simulink model "sm_stewart_platform"  (R2019b)
settings: Solver=ode45  StartTime=0.0  StopTime=450  MaxStep=0.2  RelTol=1e-3  EnableMultiTasking=on
model workspace (MAT data in the model file):
  g_density = 5
values from neighbouring files (symbols this model uses):
  B = base_points.Data(:,:,1)    [run_this_for_sim.m]
  base_radius = 0.75*100    (= 75)    [run_this_for_sim.m]
  desired_max_angle = 10    [run_this_for_sim.m]
  desired_max_x = 0.05    [run_this_for_sim.m]
  desired_max_y = desired_max_x    (= 0.05)    [run_this_for_sim.m]
  desired_max_z = 0.05    [run_this_for_sim.m]
  initial_integral_force = 200    [run_this_for_sim.m]
  leg_max = leg_min+0.3    (= 1.322)    [run_this_for_sim.m]
  leg_min = 1.022    [run_this_for_sim.m]
  leg_thickness = 75/1000    (= 0.075)    [run_this_for_sim.m]
  lower_leg_length = upper_leg_length    (= 0.511)    [run_this_for_sim.m]
  max_velocity = 0.15    [run_this_for_sim.m]
  P = platform_points.Data(:,:,1)    [run_this_for_sim.m]
  platform_radius = 0.75*base_radius    (= 56.25)    [run_this_for_sim.m]
  platform_thickness = 0.1/8    (= 0.0125)    [run_this_for_sim.m]
  trajectory_smoothing = 1/1.5    (= 0.666666666667)    [run_this_for_sim.m]
  upper_leg_length = dead_length/2    (= 0.511)    [run_this_for_sim.m]
  work_height = 1.2*100    (= 120)    [run_this_for_sim.m]
undefined symbols (not defined in the file or in its folder): nom_length, X, Z
libraries: sp_lib x18, nesl_utility x11, sm_lib x9, simulink x2
(part 9 of 10)

== system sm_stewart_platform/Stewart Platform System/Manipulator/Platform ==
  Bus Creator : BusCreator  Inputs=6
  Coupling Transform : sm_lib/Frames and Transforms/Rigid Transform  TranslationMethod=StandardAxis  TranslationStandardOffset=(1 - 2 * kind_val) * (hex_thick / 2 + flange_len)  TranslationLengthUnit=cm  TranslationStandardAxis=+Z  TranslationCartesianOffset=[0 0 0]  TranslationROffset=0  TranslationROffsetUnits=m  TranslationZOffset=0  TranslationZOffsetUnits=m  TranslationThetaOffset=0  TranslationThetaOffsetUnits=deg  RotationMethod=AlignedAxes  RotationAngleUnits=deg  RotationStandardAxis=+Z  RotationAngle=0  RotationArbitraryAxis=[0 0 1]  FollAlignAxisA=+Z  BaseAlignAxisA=+X  FollAlignAxisB=+X  BaseAlignAxisB=+Z  RotationSequenceAxes=FollowerAxes  RotationSequence=XYX  RotationSequenceAngles=[0 0 0]  RotationSequenceAnglesUnits=deg  RotationMatrix=[1 0 0; 0 1 0; 0 0 1]
  Plate Coupling 1 : sp_lib/Plate Coupling 1  index=0 + kind_val  hex_rad=hex_rad  hex_skew=hex_skew  flange_width=flange_width  flange_thick=flange_thick  flange_sep=flange_sep  flange_ref_rot=kind_val * 180
  Plate Coupling 2 : sp_lib/Plate Coupling 1  index=1 + kind_val  hex_rad=hex_rad  hex_skew=hex_skew  flange_width=flange_width  flange_thick=flange_thick  flange_sep=flange_sep  flange_ref_rot=kind_val * 180
  Plate Coupling 3 : sp_lib/Plate Coupling 1  index=2 + kind_val  hex_rad=hex_rad  hex_skew=hex_skew  flange_width=flange_width  flange_thick=flange_thick  flange_sep=flange_sep  flange_ref_rot=kind_val * 180
  Plate Coupling 4 : sp_lib/Plate Coupling 1  index=3 + kind_val  hex_rad=hex_rad  hex_skew=hex_skew  flange_width=flange_width  flange_thick=flange_thick  flange_sep=flange_sep  flange_ref_rot=kind_val * 180
  Plate Coupling 5 : sp_lib/Plate Coupling 1  index=4 + kind_val  hex_rad=hex_rad  hex_skew=hex_skew  flange_width=flange_width  flange_thick=flange_thick  flange_sep=flange_sep  flange_ref_rot=kind_val * 180
  Plate Coupling 6 : sp_lib/Plate Coupling 1  index=5 + kind_val  hex_rad=hex_rad  hex_skew=hex_skew  flange_width=flange_width  flange_thick=flange_thick  flange_sep=flange_sep  flange_ref_rot=kind_val * 180
  Reference Frame : sm_lib/Frames and Transforms/Reference Frame
  Skewed Hexagon : Subsystem  mask(Skewed Hexagon){rad=hex_rad, thick=hex_thick, skew=hex_skew, diffuse=diffuse, specualr=specular, shininess=shininess}
      mask prompts: rad "Radius (cm)"; thick "Thickness (cm)"; diffuse "Diffuse (rgba)"; specualr "Specular (rgba)"; shininess "Shininess (0-128)"
      mask help:
      | Models a hexagonal prism with 3-fold symmetry.
      |
      | A skew factor in the range (-0.5, +0.5) controls the shape of the hexagon.  A zero skew factor produces a regular hexagon cross section, and values toward +/- 0.5 produce progressively more triangular hexagons.
      mask init:
      | angles = pi/3 * ((0:1:5) + skew * [+1 -1 +1 -1 +1 -1]);
      | cross_sect = rad * [cos(angles); sin(angles)]';
      mask Help:
      | A <em>Skewed Hexagon</em> models a hexagonal prism with 3-fold symmetry.
      | 
      | A skew factor in the range (-0.5, +0.5) controls the shape of the hexagon.  A zero
      | skew factor produces a regular hexagon cross section, and values toward +/- 0.5
      | produce progressively more triangular hexagons.
      | 
      | See <em>Skewed Hexagons</em> in the documentation of the <em>Hexagon Plate</em>
      | block for more details.
      | 
      | <h3>Geometry</h3>
      | 
      | The <em>Geom</em> tab parameters specify the geometry of the skewed hexagon.
      | 
      | <ul>
      | 
      | <li> <b>Radius</b> The radius of thee circle on which the vertices of
      |   the hexagonal cross section lie.
      | 
      | <li> <b> Thickness</b> The thickness (length) of the hexagonal prism.
      | 
      | <li> <b>Skew</b> The skew factor of the hexagonal cross section, in the
      |   range (-0.5, +0.5).
      | 
      | </ul>
      | 
      | <h3>Visualization</h3>
      | 
      | The <em>Graphics</em> tab parameters specify the visualization aspects of the skewed
      | hexagon.
      | 
      | 
      | <ul>
      | 
      | <li> <b>Diffuse</b> The diffuse color of the skewed hexagon.  This is an RGB
      | 3-vector or an RGBA 4-vector with all components in the range [0, 1].
      | 
      | <li> <b>Specular</b> The specular color of the skewed hexagon.  This is an RGB
      | 3-vector or an RGBA 4-vector with all components in the range [0, 1].
      | 
      | <li> <b>Shininess</b> The shininess of the skewed hexagon.  This is a scalar
      | value in the range [0, 128].
      | 
      | </ul>
      | 
      | 
      | <h3>Ports</h3>
      | 
      | <ul>
      | 
      | <li> <b>ref</b> Reference frame of the skewed hexagon.  The origin of this frame
      |   is located at the center of the hexagonal prism, and the z-axis is aligned
      |   with the axis of the prism.
      | 
      | </ul>
      mask Display:
      | image(imread('sm_stewart_platform_skewedhexagon.png'))
      | color('white')
      | port_label('RConn', 1, 'ref')
  ref : PMIOPort  Side=Left
  leg1 : PMIOPort  Port=2  Side=Right
  leg2 : PMIOPort  Port=3  Side=Right
  leg3 : PMIOPort  Port=4  Side=Right
  leg4 : PMIOPort  Port=5  Side=Right
  leg5 : PMIOPort  Port=6  Side=Right
  leg6 : PMIOPort  Port=7  Side=Right
  plat_ang : Outport  VectorParamsAs1DForOutWhenUnconnected=off
  wires:
  Plate Coupling 6/1 -> Bus Creator/1
  Plate Coupling 5/1 -> Bus Creator/2
  Plate Coupling 4/1 -> Bus Creator/3
  Plate Coupling 3/1 -> Bus Creator/4
  Plate Coupling 2/1 -> Bus Creator/5
  Plate Coupling 1/1 -> Bus Creator/6
  Bus Creator/1 -> plat_ang/1
  connections:
  Plate Coupling 6/RConn1 -- leg6/RConn1
  Plate Coupling 5/RConn1 -- leg5/RConn1
  Plate Coupling 4/RConn1 -- leg4/RConn1
  Plate Coupling 3/RConn1 -- leg3/RConn1
  Plate Coupling 2/RConn1 -- leg2/RConn1
  Plate Coupling 1/RConn1 -- leg1/RConn1
  Plate Coupling 5/LConn1 -- Plate Coupling 6/LConn1 -- Coupling Transform/RConn1 -- Plate Coupling 4/LConn1 -- Plate Coupling 3/LConn1 -- Plate Coupling 2/LConn1 -- Plate Coupling 1/LConn1
  Coupling Transform/LConn1 -- Skewed Hexagon/RConn1 -- ref/RConn1 -- Reference Frame/RConn1

== system sm_stewart_platform/Subsystem/Reference Trajectory Generator/Euler XYZ ==
  angles : Inport
  11 : Fcn  Expr=cos(u[2])*cos(u[3])
  12 : Fcn  Expr=-cos(u[2])*sin(u[3])
  13 : Fcn  Expr=sin(u[2])
  21 : Fcn  Expr=cos(u[3])*sin(u[2])*sin(u[1])+cos(u[1])*sin(u[3])
  22 : Fcn  Expr=cos(u[1])*cos(u[3]) - sin(u[1])*sin(u[2])*sin(u[3])
  23 : Fcn  Expr=-sin(u[1])*cos(u[2])
  31 : Fcn  Expr=sin(u[1])*sin(u[3]) - cos(u[1])*cos(u[3])*sin(u[2])
  32 : Fcn  Expr=cos(u[3])*sin(u[1])+cos(u[1])*sin(u[2])*sin(u[3])
  33 : Fcn  Expr=cos(u[1])*cos(u[2])
  Mux2 : Mux  Inputs=9
  Reshape 9x1->3x3 : Reshape  OutputDimensionality=Customize  OutputDimensions=[3,3]
  R : Outport  VectorParamsAs1DForOutWhenUnconnected=off
  wires:
  angles/1 -> 23/1, 33/1, 13/1, 32/1, 22/1, 12/1, 31/1, 21/1, 11/1
  33/1 -> Mux2/9
  23/1 -> Mux2/8
  13/1 -> Mux2/7
  32/1 -> Mux2/6
  22/1 -> Mux2/5
  12/1 -> Mux2/4
  31/1 -> Mux2/3
  21/1 -> Mux2/2
  11/1 -> Mux2/1
  Mux2/1 -> Reshape 9x1->3x3/1
  Reshape 9x1->3x3/1 -> R/1

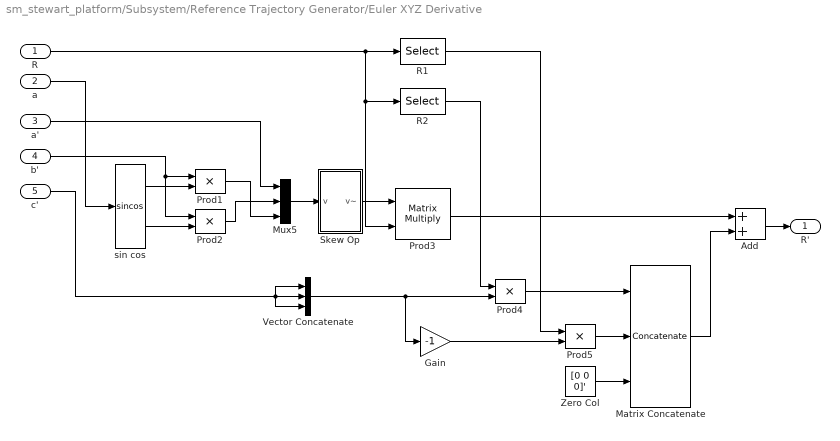
== system sm_stewart_platform/Subsystem/Reference Trajectory Generator/Euler XYZ Derivative ==
  R : Inport
  a : Inport  Port=2
  a' : Inport  Port=3
  b' : Inport  Port=4
  c' : Inport  Port=5
  Add : Sum
  Gain : Gain  Gain=-1
  Matrix Concatenate : Concatenate  NumInputs=3  Mode=Multidimensional array  ConcatenateDimension=2
  Mux5 : Mux  Inputs=3
  Prod{1..2,4..5} (4 alike) : Product  RndMeth=Zero
  Prod3 : Product  Multiplication=Matrix(*)  RndMeth=Zero
  R1 : Selector  NumberOfDimensions=2  InputPortWidth=3  IndexOptions=Select all,Index vector (dialog)  Indices=[1 3],1  OutputSizes=1,1
  R2 : Selector  NumberOfDimensions=2  InputPortWidth=3  IndexOptions=Select all,Index vector (dialog)  Indices=[1 3],2  OutputSizes=1,1
  Skew Op : Subsystem
  Vector Concatenate : Concatenate  NumInputs=3  Mode=Multidimensional array
  Zero Col : Constant  Value=[0 0 0]'
  sin cos : Trigonometry  Operator=sincos
  R' : Outport  VectorParamsAs1DForOutWhenUnconnected=off
  wires:
  a/1 -> sin cos/1
  sin cos/1 -> Prod1/2
  sin cos/2 -> Prod2/2
  b'/1 -> Prod2/1, Prod1/1
  a'/1 -> Mux5/1
  Prod2/1 -> Mux5/2
  Prod1/1 -> Mux5/3
  Mux5/1 -> Skew Op/1(v)
  Vector Concatenate/1 -> Prod4/2, Gain/1
  R2/1 -> Prod4/1
  Gain/1 -> Prod5/2
  Zero Col/1 -> Matrix Concatenate/3
  Prod5/1 -> Matrix Concatenate/2
  Prod4/1 -> Matrix Concatenate/1
  R1/1 -> Prod5/1
  Prod3/1 -> Add/1
  Matrix Concatenate/1 -> Add/2
  Add/1 -> R'/1
  R/1 -> R1/1, Prod3/2, R2/1
  Skew Op/1(v~) -> Prod3/1
  c'/1 -> Vector Concatenate/2, Vector Concatenate/1, Vector Concatenate/3

== system sm_stewart_platform/Subsystem/Reference Trajectory Generator/Rx sinusoid ==
  t : Inport
  Add : Sum  Inputs=|++
  Add2 : Sum  Inputs=++|
  amp1 : Gain  Gain=A
  amp2 : Gain  Gain=w*A*pi/180
  deg2rad : Gain  Gain=pi/180
  freq : Gain  Gain=w
  offset : Constant  Value=k  VectorParams1D=off
  phase : Constant  Value=p  VectorParams1D=off
  sin cos : Trigonometry  Operator=sincos
  f : Outport  VectorParamsAs1DForOutWhenUnconnected=off
  f' : Outport  Port=2  VectorParamsAs1DForOutWhenUnconnected=off
  wires:
  t/1 -> freq/1
  Add/1 -> deg2rad/1
  phase/1 -> Add/2
  amp2/1 -> f'/1
  Add2/1 -> f/1
  offset/1 -> Add2/1
  sin cos/1 -> amp1/1
  sin cos/2 -> amp2/1
  amp1/1 -> Add2/2
  freq/1 -> Add/1
  deg2rad/1 -> sin cos/1

== system sm_stewart_platform/Subsystem/Reference Trajectory Generator/Ry sinusoid ==
  t : Inport
  Add : Sum  Inputs=|++
  Add2 : Sum  Inputs=++|
  amp1 : Gain  Gain=A
  amp2 : Gain  Gain=w*A*pi/180
  deg2rad : Gain  Gain=pi/180
  freq : Gain  Gain=w
  offset : Constant  Value=k  VectorParams1D=off
  phase : Constant  Value=p  VectorParams1D=off
  sin cos : Trigonometry  Operator=sincos
  f : Outport  VectorParamsAs1DForOutWhenUnconnected=off
  f' : Outport  Port=2  VectorParamsAs1DForOutWhenUnconnected=off
  wires:
  t/1 -> freq/1
  Add/1 -> deg2rad/1
  phase/1 -> Add/2
  amp2/1 -> f'/1
  Add2/1 -> f/1
  offset/1 -> Add2/1
  sin cos/1 -> amp1/1
  sin cos/2 -> amp2/1
  amp1/1 -> Add2/2
  freq/1 -> Add/1
  deg2rad/1 -> sin cos/1

== system sm_stewart_platform/Subsystem/Reference Trajectory Generator/Rz sinusoid ==
  t : Inport
  Add : Sum  Inputs=|++
  Add2 : Sum  Inputs=++|
  amp1 : Gain  Gain=A
  amp2 : Gain  Gain=w*A*pi/180
  deg2rad : Gain  Gain=pi/180
  freq : Gain  Gain=w
  offset : Constant  Value=k  VectorParams1D=off
  phase : Constant  Value=p  VectorParams1D=off
  sin cos : Trigonometry  Operator=sincos
  f : Outport  VectorParamsAs1DForOutWhenUnconnected=off
  f' : Outport  Port=2  VectorParamsAs1DForOutWhenUnconnected=off
  wires:
  t/1 -> freq/1
  Add/1 -> deg2rad/1
  phase/1 -> Add/2
  amp2/1 -> f'/1
  Add2/1 -> f/1
  offset/1 -> Add2/1
  sin cos/1 -> amp1/1
  sin cos/2 -> amp2/1
  amp1/1 -> Add2/2
  freq/1 -> Add/1
  deg2rad/1 -> sin cos/1

== system sm_stewart_platform/Subsystem/Reference Trajectory Generator/dx sinusoid ==
  t : Inport
  Add : Sum  Inputs=|++
  Add2 : Sum  Inputs=++|
  amp1 : Gain  Gain=A
  amp2 : Gain  Gain=w*A*pi/180
  deg2rad : Gain  Gain=pi/180
  freq : Gain  Gain=w
  offset : Constant  Value=k  VectorParams1D=off
  phase : Constant  Value=p  VectorParams1D=off
  sin cos : Trigonometry  Operator=sincos
  f : Outport  VectorParamsAs1DForOutWhenUnconnected=off
  f' : Outport  Port=2  VectorParamsAs1DForOutWhenUnconnected=off
  wires:
  t/1 -> freq/1
  Add/1 -> deg2rad/1
  phase/1 -> Add/2
  amp2/1 -> f'/1
  Add2/1 -> f/1
  offset/1 -> Add2/1
  sin cos/1 -> amp1/1
  sin cos/2 -> amp2/1
  amp1/1 -> Add2/2
  freq/1 -> Add/1
  deg2rad/1 -> sin cos/1

== system sm_stewart_platform/Subsystem/Reference Trajectory Generator/dy sinusoid ==
  t : Inport
  Add : Sum  Inputs=|++
  Add2 : Sum  Inputs=++|
  amp1 : Gain  Gain=A
  amp2 : Gain  Gain=w*A*pi/180
  deg2rad : Gain  Gain=pi/180
  freq : Gain  Gain=w
  offset : Constant  Value=k  VectorParams1D=off
  phase : Constant  Value=p  VectorParams1D=off
  sin cos : Trigonometry  Operator=sincos
  f : Outport  VectorParamsAs1DForOutWhenUnconnected=off
  f' : Outport  Port=2  VectorParamsAs1DForOutWhenUnconnected=off
  wires:
  t/1 -> freq/1
  Add/1 -> deg2rad/1
  phase/1 -> Add/2
  amp2/1 -> f'/1
  Add2/1 -> f/1
  offset/1 -> Add2/1
  sin cos/1 -> amp1/1
  sin cos/2 -> amp2/1
  amp1/1 -> Add2/2
  freq/1 -> Add/1
  deg2rad/1 -> sin cos/1

== system sm_stewart_platform/Subsystem/Reference Trajectory Generator/dz sinusoid ==
  t : Inport
  Add : Sum  Inputs=|++
  Add2 : Sum  Inputs=++|
  amp1 : Gain  Gain=A
  amp2 : Gain  Gain=w*A*pi/180
  deg2rad : Gain  Gain=pi/180
  freq : Gain  Gain=w
  offset : Constant  Value=k  VectorParams1D=off
  phase : Constant  Value=p  VectorParams1D=off
  sin cos : Trigonometry  Operator=sincos
  f : Outport  VectorParamsAs1DForOutWhenUnconnected=off
  f' : Outport  Port=2  VectorParamsAs1DForOutWhenUnconnected=off
  wires:
  t/1 -> freq/1
  Add/1 -> deg2rad/1
  phase/1 -> Add/2
  amp2/1 -> f'/1
  Add2/1 -> f/1
  offset/1 -> Add2/1
  sin cos/1 -> amp1/1
  sin cos/2 -> amp2/1
  amp1/1 -> Add2/2
  freq/1 -> Add/1
  deg2rad/1 -> sin cos/1

== system sm_stewart_platform/Subsystem/Reference Trajectory Generator1/Euler XYZ ==
  angles : Inport
  11 : Fcn  Expr=cos(u[2])*cos(u[3])
  12 : Fcn  Expr=-cos(u[2])*sin(u[3])
  13 : Fcn  Expr=sin(u[2])
  21 : Fcn  Expr=cos(u[3])*sin(u[2])*sin(u[1])+cos(u[1])*sin(u[3])
  22 : Fcn  Expr=cos(u[1])*cos(u[3]) - sin(u[1])*sin(u[2])*sin(u[3])
  23 : Fcn  Expr=-sin(u[1])*cos(u[2])
  31 : Fcn  Expr=sin(u[1])*sin(u[3]) - cos(u[1])*cos(u[3])*sin(u[2])
  32 : Fcn  Expr=cos(u[3])*sin(u[1])+cos(u[1])*sin(u[2])*sin(u[3])
  33 : Fcn  Expr=cos(u[1])*cos(u[2])
  Mux2 : Mux  Inputs=9
  Reshape 9x1->3x3 : Reshape  OutputDimensionality=Customize  OutputDimensions=[3,3]
  R : Outport  VectorParamsAs1DForOutWhenUnconnected=off
  wires:
  angles/1 -> 23/1, 33/1, 13/1, 32/1, 22/1, 12/1, 31/1, 21/1, 11/1
  33/1 -> Mux2/9
  23/1 -> Mux2/8
  13/1 -> Mux2/7
  32/1 -> Mux2/6
  22/1 -> Mux2/5
  12/1 -> Mux2/4
  31/1 -> Mux2/3
  21/1 -> Mux2/2
  11/1 -> Mux2/1
  Mux2/1 -> Reshape 9x1->3x3/1
  Reshape 9x1->3x3/1 -> R/1

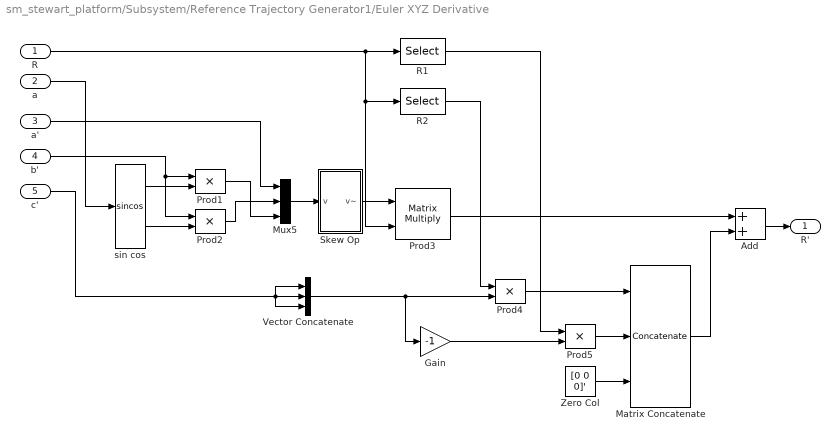
== system sm_stewart_platform/Subsystem/Reference Trajectory Generator1/Euler XYZ Derivative ==
  R : Inport
  a : Inport  Port=2
  a' : Inport  Port=3
  b' : Inport  Port=4
  c' : Inport  Port=5
  Add : Sum
  Gain : Gain  Gain=-1
  Matrix Concatenate : Concatenate  NumInputs=3  Mode=Multidimensional array  ConcatenateDimension=2
  Mux5 : Mux  Inputs=3
  Prod{1..2,4..5} (4 alike) : Product  RndMeth=Zero
  Prod3 : Product  Multiplication=Matrix(*)  RndMeth=Zero
  R1 : Selector  NumberOfDimensions=2  InputPortWidth=3  IndexOptions=Select all,Index vector (dialog)  Indices=[1 3],1  OutputSizes=1,1
  R2 : Selector  NumberOfDimensions=2  InputPortWidth=3  IndexOptions=Select all,Index vector (dialog)  Indices=[1 3],2  OutputSizes=1,1
  Skew Op : Subsystem
  Vector Concatenate : Concatenate  NumInputs=3  Mode=Multidimensional array
  Zero Col : Constant  Value=[0 0 0]'
  sin cos : Trigonometry  Operator=sincos
  R' : Outport  VectorParamsAs1DForOutWhenUnconnected=off
  wires:
  a/1 -> sin cos/1
  sin cos/1 -> Prod1/2
  sin cos/2 -> Prod2/2
  b'/1 -> Prod2/1, Prod1/1
  a'/1 -> Mux5/1
  Prod2/1 -> Mux5/2
  Prod1/1 -> Mux5/3
  Mux5/1 -> Skew Op/1(v)
  Vector Concatenate/1 -> Prod4/2, Gain/1
  R2/1 -> Prod4/1
  Gain/1 -> Prod5/2
  Zero Col/1 -> Matrix Concatenate/3
  Prod5/1 -> Matrix Concatenate/2
  Prod4/1 -> Matrix Concatenate/1
  R1/1 -> Prod5/1
  Prod3/1 -> Add/1
  Matrix Concatenate/1 -> Add/2
  Add/1 -> R'/1
  R/1 -> R1/1, Prod3/2, R2/1
  Skew Op/1(v~) -> Prod3/1
  c'/1 -> Vector Concatenate/2, Vector Concatenate/1, Vector Concatenate/3

== system sm_stewart_platform/Subsystem/Reference Trajectory Generator1/Rx sinusoid ==
  t : Inport
  Add : Sum  Inputs=|++
  Add2 : Sum  Inputs=++|
  amp1 : Gain  Gain=A
  amp2 : Gain  Gain=w*A*pi/180
  deg2rad : Gain  Gain=pi/180
  freq : Gain  Gain=w
  offset : Constant  Value=k  VectorParams1D=off
  phase : Constant  Value=p  VectorParams1D=off
  sin cos : Trigonometry  Operator=sincos
  f : Outport  VectorParamsAs1DForOutWhenUnconnected=off
  f' : Outport  Port=2  VectorParamsAs1DForOutWhenUnconnected=off
  wires:
  t/1 -> freq/1
  Add/1 -> deg2rad/1
  phase/1 -> Add/2
  amp2/1 -> f'/1
  Add2/1 -> f/1
  offset/1 -> Add2/1
  sin cos/1 -> amp1/1
  sin cos/2 -> amp2/1
  amp1/1 -> Add2/2
  freq/1 -> Add/1
  deg2rad/1 -> sin cos/1

== system sm_stewart_platform/Subsystem/Reference Trajectory Generator1/Ry sinusoid ==
  t : Inport
  Add : Sum  Inputs=|++
  Add2 : Sum  Inputs=++|
  amp1 : Gain  Gain=A
  amp2 : Gain  Gain=w*A*pi/180
  deg2rad : Gain  Gain=pi/180
  freq : Gain  Gain=w
  offset : Constant  Value=k  VectorParams1D=off
  phase : Constant  Value=p  VectorParams1D=off
  sin cos : Trigonometry  Operator=sincos
  f : Outport  VectorParamsAs1DForOutWhenUnconnected=off
  f' : Outport  Port=2  VectorParamsAs1DForOutWhenUnconnected=off
  wires:
  t/1 -> freq/1
  Add/1 -> deg2rad/1
  phase/1 -> Add/2
  amp2/1 -> f'/1
  Add2/1 -> f/1
  offset/1 -> Add2/1
  sin cos/1 -> amp1/1
  sin cos/2 -> amp2/1
  amp1/1 -> Add2/2
  freq/1 -> Add/1
  deg2rad/1 -> sin cos/1

== system sm_stewart_platform/Subsystem/Reference Trajectory Generator1/Rz sinusoid ==
  t : Inport
  Add : Sum  Inputs=|++
  Add2 : Sum  Inputs=++|
  amp1 : Gain  Gain=A
  amp2 : Gain  Gain=w*A*pi/180
  deg2rad : Gain  Gain=pi/180
  freq : Gain  Gain=w
  offset : Constant  Value=k  VectorParams1D=off
  phase : Constant  Value=p  VectorParams1D=off
  sin cos : Trigonometry  Operator=sincos
  f : Outport  VectorParamsAs1DForOutWhenUnconnected=off
  f' : Outport  Port=2  VectorParamsAs1DForOutWhenUnconnected=off
  wires:
  t/1 -> freq/1
  Add/1 -> deg2rad/1
  phase/1 -> Add/2
  amp2/1 -> f'/1
  Add2/1 -> f/1
  offset/1 -> Add2/1
  sin cos/1 -> amp1/1
  sin cos/2 -> amp2/1
  amp1/1 -> Add2/2
  freq/1 -> Add/1
  deg2rad/1 -> sin cos/1

== system sm_stewart_platform/Subsystem/Reference Trajectory Generator1/dx sinusoid ==
  t : Inport
  Add : Sum  Inputs=|++
  Add2 : Sum  Inputs=++|
  amp1 : Gain  Gain=A
  amp2 : Gain  Gain=w*A*pi/180
  deg2rad : Gain  Gain=pi/180
  freq : Gain  Gain=w
  offset : Constant  Value=k  VectorParams1D=off
  phase : Constant  Value=p  VectorParams1D=off
  sin cos : Trigonometry  Operator=sincos
  f : Outport  VectorParamsAs1DForOutWhenUnconnected=off
  f' : Outport  Port=2  VectorParamsAs1DForOutWhenUnconnected=off
  wires:
  t/1 -> freq/1
  Add/1 -> deg2rad/1
  phase/1 -> Add/2
  amp2/1 -> f'/1
  Add2/1 -> f/1
  offset/1 -> Add2/1
  sin cos/1 -> amp1/1
  sin cos/2 -> amp2/1
  amp1/1 -> Add2/2
  freq/1 -> Add/1
  deg2rad/1 -> sin cos/1

== system sm_stewart_platform/Subsystem/Reference Trajectory Generator1/dy sinusoid ==
  t : Inport
  Add : Sum  Inputs=|++
  Add2 : Sum  Inputs=++|
  amp1 : Gain  Gain=A
  amp2 : Gain  Gain=w*A*pi/180
  deg2rad : Gain  Gain=pi/180
  freq : Gain  Gain=w
  offset : Constant  Value=k  VectorParams1D=off
  phase : Constant  Value=p  VectorParams1D=off
  sin cos : Trigonometry  Operator=sincos
  f : Outport  VectorParamsAs1DForOutWhenUnconnected=off
  f' : Outport  Port=2  VectorParamsAs1DForOutWhenUnconnected=off
  wires:
  t/1 -> freq/1
  Add/1 -> deg2rad/1
  phase/1 -> Add/2
  amp2/1 -> f'/1
  Add2/1 -> f/1
  offset/1 -> Add2/1
  sin cos/1 -> amp1/1
  sin cos/2 -> amp2/1
  amp1/1 -> Add2/2
  freq/1 -> Add/1
  deg2rad/1 -> sin cos/1

== system sm_stewart_platform/Subsystem/Reference Trajectory Generator1/dz sinusoid ==
  t : Inport
  Add : Sum  Inputs=|++
  Add2 : Sum  Inputs=++|
  amp1 : Gain  Gain=A
  amp2 : Gain  Gain=w*A*pi/180
  deg2rad : Gain  Gain=pi/180
  freq : Gain  Gain=w
  offset : Constant  Value=k  VectorParams1D=off
  phase : Constant  Value=p  VectorParams1D=off
  sin cos : Trigonometry  Operator=sincos
  f : Outport  VectorParamsAs1DForOutWhenUnconnected=off
  f' : Outport  Port=2  VectorParamsAs1DForOutWhenUnconnected=off
  wires:
  t/1 -> freq/1
  Add/1 -> deg2rad/1
  phase/1 -> Add/2
  amp2/1 -> f'/1
  Add2/1 -> f/1
  offset/1 -> Add2/1
  sin cos/1 -> amp1/1
  sin cos/2 -> amp2/1
  amp1/1 -> Add2/2
  freq/1 -> Add/1
  deg2rad/1 -> sin cos/1

== system sm_stewart_platform/Subsystem/Reference Trajectory Generator2/Euler XYZ ==
  angles : Inport
  11 : Fcn  Expr=cos(u[2])*cos(u[3])
  12 : Fcn  Expr=-cos(u[2])*sin(u[3])
  13 : Fcn  Expr=sin(u[2])
  21 : Fcn  Expr=cos(u[3])*sin(u[2])*sin(u[1])+cos(u[1])*sin(u[3])
  22 : Fcn  Expr=cos(u[1])*cos(u[3]) - sin(u[1])*sin(u[2])*sin(u[3])
  23 : Fcn  Expr=-sin(u[1])*cos(u[2])
  31 : Fcn  Expr=sin(u[1])*sin(u[3]) - cos(u[1])*cos(u[3])*sin(u[2])
  32 : Fcn  Expr=cos(u[3])*sin(u[1])+cos(u[1])*sin(u[2])*sin(u[3])
  33 : Fcn  Expr=cos(u[1])*cos(u[2])
  Mux2 : Mux  Inputs=9
  Reshape 9x1->3x3 : Reshape  OutputDimensionality=Customize  OutputDimensions=[3,3]
  R : Outport  VectorParamsAs1DForOutWhenUnconnected=off
  wires:
  angles/1 -> 23/1, 33/1, 13/1, 32/1, 22/1, 12/1, 31/1, 21/1, 11/1
  33/1 -> Mux2/9
  23/1 -> Mux2/8
  13/1 -> Mux2/7
  32/1 -> Mux2/6
  22/1 -> Mux2/5
  12/1 -> Mux2/4
  31/1 -> Mux2/3
  21/1 -> Mux2/2
  11/1 -> Mux2/1
  Mux2/1 -> Reshape 9x1->3x3/1
  Reshape 9x1->3x3/1 -> R/1

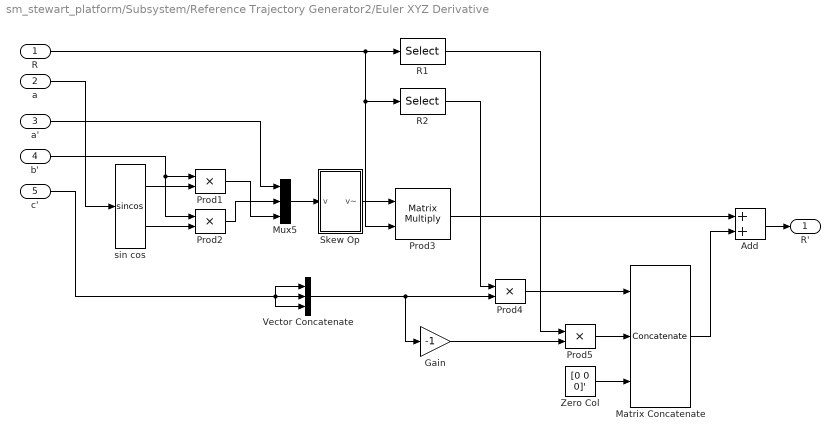
== system sm_stewart_platform/Subsystem/Reference Trajectory Generator2/Euler XYZ Derivative ==
  R : Inport
  a : Inport  Port=2
  a' : Inport  Port=3
  b' : Inport  Port=4
  c' : Inport  Port=5
  Add : Sum
  Gain : Gain  Gain=-1
  Matrix Concatenate : Concatenate  NumInputs=3  Mode=Multidimensional array  ConcatenateDimension=2
  Mux5 : Mux  Inputs=3
  Prod{1..2,4..5} (4 alike) : Product  RndMeth=Zero
  Prod3 : Product  Multiplication=Matrix(*)  RndMeth=Zero
  R1 : Selector  NumberOfDimensions=2  InputPortWidth=3  IndexOptions=Select all,Index vector (dialog)  Indices=[1 3],1  OutputSizes=1,1
  R2 : Selector  NumberOfDimensions=2  InputPortWidth=3  IndexOptions=Select all,Index vector (dialog)  Indices=[1 3],2  OutputSizes=1,1
  Skew Op : Subsystem
  Vector Concatenate : Concatenate  NumInputs=3  Mode=Multidimensional array
  Zero Col : Constant  Value=[0 0 0]'
  sin cos : Trigonometry  Operator=sincos
  R' : Outport  VectorParamsAs1DForOutWhenUnconnected=off
  wires:
  a/1 -> sin cos/1
  sin cos/1 -> Prod1/2
  sin cos/2 -> Prod2/2
  b'/1 -> Prod2/1, Prod1/1
  a'/1 -> Mux5/1
  Prod2/1 -> Mux5/2
  Prod1/1 -> Mux5/3
  Mux5/1 -> Skew Op/1(v)
  Vector Concatenate/1 -> Prod4/2, Gain/1
  R2/1 -> Prod4/1
  Gain/1 -> Prod5/2
  Zero Col/1 -> Matrix Concatenate/3
  Prod5/1 -> Matrix Concatenate/2
  Prod4/1 -> Matrix Concatenate/1
  R1/1 -> Prod5/1
  Prod3/1 -> Add/1
  Matrix Concatenate/1 -> Add/2
  Add/1 -> R'/1
  R/1 -> R1/1, Prod3/2, R2/1
  Skew Op/1(v~) -> Prod3/1
  c'/1 -> Vector Concatenate/2, Vector Concatenate/1, Vector Concatenate/3

== system sm_stewart_platform/Subsystem/Reference Trajectory Generator2/Rx sinusoid ==
  t : Inport
  Add : Sum  Inputs=|++
  Add2 : Sum  Inputs=++|
  amp1 : Gain  Gain=A
  amp2 : Gain  Gain=w*A*pi/180
  deg2rad : Gain  Gain=pi/180
  freq : Gain  Gain=w
  offset : Constant  Value=k  VectorParams1D=off
  phase : Constant  Value=p  VectorParams1D=off
  sin cos : Trigonometry  Operator=sincos
  f : Outport  VectorParamsAs1DForOutWhenUnconnected=off
  f' : Outport  Port=2  VectorParamsAs1DForOutWhenUnconnected=off
  wires:
  t/1 -> freq/1
  Add/1 -> deg2rad/1
  phase/1 -> Add/2
  amp2/1 -> f'/1
  Add2/1 -> f/1
  offset/1 -> Add2/1
  sin cos/1 -> amp1/1
  sin cos/2 -> amp2/1
  amp1/1 -> Add2/2
  freq/1 -> Add/1
  deg2rad/1 -> sin cos/1

== system sm_stewart_platform/Subsystem/Reference Trajectory Generator2/Ry sinusoid ==
  t : Inport
  Add : Sum  Inputs=|++
  Add2 : Sum  Inputs=++|
  amp1 : Gain  Gain=A
  amp2 : Gain  Gain=w*A*pi/180
  deg2rad : Gain  Gain=pi/180
  freq : Gain  Gain=w
  offset : Constant  Value=k  VectorParams1D=off
  phase : Constant  Value=p  VectorParams1D=off
  sin cos : Trigonometry  Operator=sincos
  f : Outport  VectorParamsAs1DForOutWhenUnconnected=off
  f' : Outport  Port=2  VectorParamsAs1DForOutWhenUnconnected=off
  wires:
  t/1 -> freq/1
  Add/1 -> deg2rad/1
  phase/1 -> Add/2
  amp2/1 -> f'/1
  Add2/1 -> f/1
  offset/1 -> Add2/1
  sin cos/1 -> amp1/1
  sin cos/2 -> amp2/1
  amp1/1 -> Add2/2
  freq/1 -> Add/1
  deg2rad/1 -> sin cos/1

== system sm_stewart_platform/Subsystem/Reference Trajectory Generator2/Rz sinusoid ==
  t : Inport
  Add : Sum  Inputs=|++
  Add2 : Sum  Inputs=++|
  amp1 : Gain  Gain=A
  amp2 : Gain  Gain=w*A*pi/180
  deg2rad : Gain  Gain=pi/180
  freq : Gain  Gain=w
  offset : Constant  Value=k  VectorParams1D=off
  phase : Constant  Value=p  VectorParams1D=off
  sin cos : Trigonometry  Operator=sincos
  f : Outport  VectorParamsAs1DForOutWhenUnconnected=off
  f' : Outport  Port=2  VectorParamsAs1DForOutWhenUnconnected=off
  wires:
  t/1 -> freq/1
  Add/1 -> deg2rad/1
  phase/1 -> Add/2
  amp2/1 -> f'/1
  Add2/1 -> f/1
  offset/1 -> Add2/1
  sin cos/1 -> amp1/1
  sin cos/2 -> amp2/1
  amp1/1 -> Add2/2
  freq/1 -> Add/1
  deg2rad/1 -> sin cos/1

== system sm_stewart_platform/Subsystem/Reference Trajectory Generator2/dx sinusoid ==
  t : Inport
  Add : Sum  Inputs=|++
  Add2 : Sum  Inputs=++|
  amp1 : Gain  Gain=A
  amp2 : Gain  Gain=w*A*pi/180
  deg2rad : Gain  Gain=pi/180
  freq : Gain  Gain=w
  offset : Constant  Value=k  VectorParams1D=off
  phase : Constant  Value=p  VectorParams1D=off
  sin cos : Trigonometry  Operator=sincos
  f : Outport  VectorParamsAs1DForOutWhenUnconnected=off
  f' : Outport  Port=2  VectorParamsAs1DForOutWhenUnconnected=off
  wires:
  t/1 -> freq/1
  Add/1 -> deg2rad/1
  phase/1 -> Add/2
  amp2/1 -> f'/1
  Add2/1 -> f/1
  offset/1 -> Add2/1
  sin cos/1 -> amp1/1
  sin cos/2 -> amp2/1
  amp1/1 -> Add2/2
  freq/1 -> Add/1
  deg2rad/1 -> sin cos/1

== system sm_stewart_platform/Subsystem/Reference Trajectory Generator2/dy sinusoid ==
  t : Inport
  Add : Sum  Inputs=|++
  Add2 : Sum  Inputs=++|
  amp1 : Gain  Gain=A
  amp2 : Gain  Gain=w*A*pi/180
  deg2rad : Gain  Gain=pi/180
  freq : Gain  Gain=w
  offset : Constant  Value=k  VectorParams1D=off
  phase : Constant  Value=p  VectorParams1D=off
  sin cos : Trigonometry  Operator=sincos
  f : Outport  VectorParamsAs1DForOutWhenUnconnected=off
  f' : Outport  Port=2  VectorParamsAs1DForOutWhenUnconnected=off
  wires:
  t/1 -> freq/1
  Add/1 -> deg2rad/1
  phase/1 -> Add/2
  amp2/1 -> f'/1
  Add2/1 -> f/1
  offset/1 -> Add2/1
  sin cos/1 -> amp1/1
  sin cos/2 -> amp2/1
  amp1/1 -> Add2/2
  freq/1 -> Add/1
  deg2rad/1 -> sin cos/1

== system sm_stewart_platform/Subsystem/Reference Trajectory Generator2/dz sinusoid ==
  t : Inport
  Add : Sum  Inputs=|++
  Add2 : Sum  Inputs=++|
  amp1 : Gain  Gain=A
  amp2 : Gain  Gain=w*A*pi/180
  deg2rad : Gain  Gain=pi/180
  freq : Gain  Gain=w
  offset : Constant  Value=k  VectorParams1D=off
  phase : Constant  Value=p  VectorParams1D=off
  sin cos : Trigonometry  Operator=sincos
  f : Outport  VectorParamsAs1DForOutWhenUnconnected=off
  f' : Outport  Port=2  VectorParamsAs1DForOutWhenUnconnected=off
  wires:
  t/1 -> freq/1
  Add/1 -> deg2rad/1
  phase/1 -> Add/2
  amp2/1 -> f'/1
  Add2/1 -> f/1
  offset/1 -> Add2/1
  sin cos/1 -> amp1/1
  sin cos/2 -> amp2/1
  amp1/1 -> Add2/2
  freq/1 -> Add/1
  deg2rad/1 -> sin cos/1

== system sm_stewart_platform/Subsystem/Reference Trajectory Generator3/Euler XYZ ==
  angles : Inport
  11 : Fcn  Expr=cos(u[2])*cos(u[3])
  12 : Fcn  Expr=-cos(u[2])*sin(u[3])
  13 : Fcn  Expr=sin(u[2])
  21 : Fcn  Expr=cos(u[3])*sin(u[2])*sin(u[1])+cos(u[1])*sin(u[3])
  22 : Fcn  Expr=cos(u[1])*cos(u[3]) - sin(u[1])*sin(u[2])*sin(u[3])
  23 : Fcn  Expr=-sin(u[1])*cos(u[2])
  31 : Fcn  Expr=sin(u[1])*sin(u[3]) - cos(u[1])*cos(u[3])*sin(u[2])
  32 : Fcn  Expr=cos(u[3])*sin(u[1])+cos(u[1])*sin(u[2])*sin(u[3])
  33 : Fcn  Expr=cos(u[1])*cos(u[2])
  Mux2 : Mux  Inputs=9
  Reshape 9x1->3x3 : Reshape  OutputDimensionality=Customize  OutputDimensions=[3,3]
  R : Outport  VectorParamsAs1DForOutWhenUnconnected=off
  wires:
  angles/1 -> 23/1, 33/1, 13/1, 32/1, 22/1, 12/1, 31/1, 21/1, 11/1
  33/1 -> Mux2/9
  23/1 -> Mux2/8
  13/1 -> Mux2/7
  32/1 -> Mux2/6
  22/1 -> Mux2/5
  12/1 -> Mux2/4
  31/1 -> Mux2/3
  21/1 -> Mux2/2
  11/1 -> Mux2/1
  Mux2/1 -> Reshape 9x1->3x3/1
  Reshape 9x1->3x3/1 -> R/1

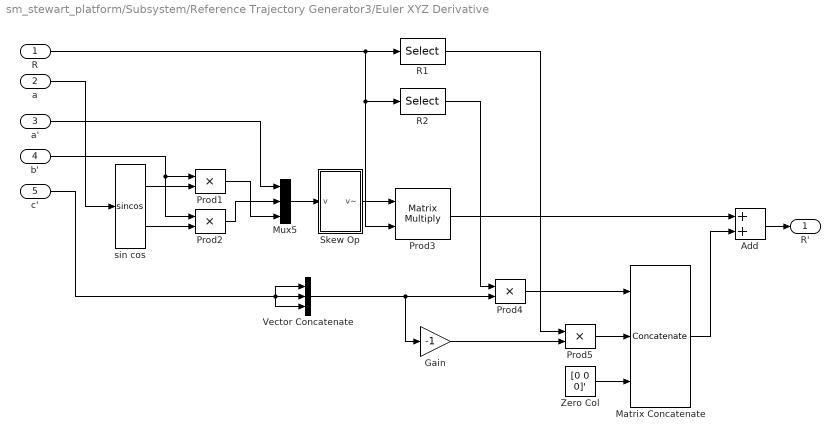
== system sm_stewart_platform/Subsystem/Reference Trajectory Generator3/Euler XYZ Derivative ==
  R : Inport
  a : Inport  Port=2
  a' : Inport  Port=3
  b' : Inport  Port=4
  c' : Inport  Port=5
  Add : Sum
  Gain : Gain  Gain=-1
  Matrix Concatenate : Concatenate  NumInputs=3  Mode=Multidimensional array  ConcatenateDimension=2
  Mux5 : Mux  Inputs=3
  Prod{1..2,4..5} (4 alike) : Product  RndMeth=Zero
  Prod3 : Product  Multiplication=Matrix(*)  RndMeth=Zero
  R1 : Selector  NumberOfDimensions=2  InputPortWidth=3  IndexOptions=Select all,Index vector (dialog)  Indices=[1 3],1  OutputSizes=1,1
  R2 : Selector  NumberOfDimensions=2  InputPortWidth=3  IndexOptions=Select all,Index vector (dialog)  Indices=[1 3],2  OutputSizes=1,1
  Skew Op : Subsystem
  Vector Concatenate : Concatenate  NumInputs=3  Mode=Multidimensional array
  Zero Col : Constant  Value=[0 0 0]'
  sin cos : Trigonometry  Operator=sincos
  R' : Outport  VectorParamsAs1DForOutWhenUnconnected=off
  wires:
  a/1 -> sin cos/1
  sin cos/1 -> Prod1/2
  sin cos/2 -> Prod2/2
  b'/1 -> Prod2/1, Prod1/1
  a'/1 -> Mux5/1
  Prod2/1 -> Mux5/2
  Prod1/1 -> Mux5/3
  Mux5/1 -> Skew Op/1(v)
  Vector Concatenate/1 -> Prod4/2, Gain/1
  R2/1 -> Prod4/1
  Gain/1 -> Prod5/2
  Zero Col/1 -> Matrix Concatenate/3
  Prod5/1 -> Matrix Concatenate/2
  Prod4/1 -> Matrix Concatenate/1
  R1/1 -> Prod5/1
  Prod3/1 -> Add/1
  Matrix Concatenate/1 -> Add/2
  Add/1 -> R'/1
  R/1 -> R1/1, Prod3/2, R2/1
  Skew Op/1(v~) -> Prod3/1
  c'/1 -> Vector Concatenate/2, Vector Concatenate/1, Vector Concatenate/3

== system sm_stewart_platform/Subsystem/Reference Trajectory Generator3/Rx sinusoid ==
  t : Inport
  Add : Sum  Inputs=|++
  Add2 : Sum  Inputs=++|
  amp1 : Gain  Gain=A
  amp2 : Gain  Gain=w*A*pi/180
  deg2rad : Gain  Gain=pi/180
  freq : Gain  Gain=w
  offset : Constant  Value=k  VectorParams1D=off
  phase : Constant  Value=p  VectorParams1D=off
  sin cos : Trigonometry  Operator=sincos
  f : Outport  VectorParamsAs1DForOutWhenUnconnected=off
  f' : Outport  Port=2  VectorParamsAs1DForOutWhenUnconnected=off
  wires:
  t/1 -> freq/1
  Add/1 -> deg2rad/1
  phase/1 -> Add/2
  amp2/1 -> f'/1
  Add2/1 -> f/1
  offset/1 -> Add2/1
  sin cos/1 -> amp1/1
  sin cos/2 -> amp2/1
  amp1/1 -> Add2/2
  freq/1 -> Add/1
  deg2rad/1 -> sin cos/1

== system sm_stewart_platform/Subsystem/Reference Trajectory Generator3/Ry sinusoid ==
  t : Inport
  Add : Sum  Inputs=|++
  Add2 : Sum  Inputs=++|
  amp1 : Gain  Gain=A
  amp2 : Gain  Gain=w*A*pi/180
  deg2rad : Gain  Gain=pi/180
  freq : Gain  Gain=w
  offset : Constant  Value=k  VectorParams1D=off
  phase : Constant  Value=p  VectorParams1D=off
  sin cos : Trigonometry  Operator=sincos
  f : Outport  VectorParamsAs1DForOutWhenUnconnected=off
  f' : Outport  Port=2  VectorParamsAs1DForOutWhenUnconnected=off
  wires:
  t/1 -> freq/1
  Add/1 -> deg2rad/1
  phase/1 -> Add/2
  amp2/1 -> f'/1
  Add2/1 -> f/1
  offset/1 -> Add2/1
  sin cos/1 -> amp1/1
  sin cos/2 -> amp2/1
  amp1/1 -> Add2/2
  freq/1 -> Add/1
  deg2rad/1 -> sin cos/1

== system sm_stewart_platform/Subsystem/Reference Trajectory Generator3/Rz sinusoid ==
  t : Inport
  Add : Sum  Inputs=|++
  Add2 : Sum  Inputs=++|
  amp1 : Gain  Gain=A
  amp2 : Gain  Gain=w*A*pi/180
  deg2rad : Gain  Gain=pi/180
  freq : Gain  Gain=w
  offset : Constant  Value=k  VectorParams1D=off
  phase : Constant  Value=p  VectorParams1D=off
  sin cos : Trigonometry  Operator=sincos
  f : Outport  VectorParamsAs1DForOutWhenUnconnected=off
  f' : Outport  Port=2  VectorParamsAs1DForOutWhenUnconnected=off
  wires:
  t/1 -> freq/1
  Add/1 -> deg2rad/1
  phase/1 -> Add/2
  amp2/1 -> f'/1
  Add2/1 -> f/1
  offset/1 -> Add2/1
  sin cos/1 -> amp1/1
  sin cos/2 -> amp2/1
  amp1/1 -> Add2/2
  freq/1 -> Add/1
  deg2rad/1 -> sin cos/1

== system sm_stewart_platform/Subsystem/Reference Trajectory Generator3/dx sinusoid ==
  t : Inport
  Add : Sum  Inputs=|++
  Add2 : Sum  Inputs=++|
  amp1 : Gain  Gain=A
  amp2 : Gain  Gain=w*A*pi/180
  deg2rad : Gain  Gain=pi/180
  freq : Gain  Gain=w
  offset : Constant  Value=k  VectorParams1D=off
  phase : Constant  Value=p  VectorParams1D=off
  sin cos : Trigonometry  Operator=sincos
  f : Outport  VectorParamsAs1DForOutWhenUnconnected=off
  f' : Outport  Port=2  VectorParamsAs1DForOutWhenUnconnected=off
  wires:
  t/1 -> freq/1
  Add/1 -> deg2rad/1
  phase/1 -> Add/2
  amp2/1 -> f'/1
  Add2/1 -> f/1
  offset/1 -> Add2/1
  sin cos/1 -> amp1/1
  sin cos/2 -> amp2/1
  amp1/1 -> Add2/2
  freq/1 -> Add/1
  deg2rad/1 -> sin cos/1

== system sm_stewart_platform/Subsystem/Reference Trajectory Generator3/dy sinusoid ==
  t : Inport
  Add : Sum  Inputs=|++
  Add2 : Sum  Inputs=++|
  amp1 : Gain  Gain=A
  amp2 : Gain  Gain=w*A*pi/180
  deg2rad : Gain  Gain=pi/180
  freq : Gain  Gain=w
  offset : Constant  Value=k  VectorParams1D=off
  phase : Constant  Value=p  VectorParams1D=off
  sin cos : Trigonometry  Operator=sincos
  f : Outport  VectorParamsAs1DForOutWhenUnconnected=off
  f' : Outport  Port=2  VectorParamsAs1DForOutWhenUnconnected=off
  wires:
  t/1 -> freq/1
  Add/1 -> deg2rad/1
  phase/1 -> Add/2
  amp2/1 -> f'/1
  Add2/1 -> f/1
  offset/1 -> Add2/1
  sin cos/1 -> amp1/1
  sin cos/2 -> amp2/1
  amp1/1 -> Add2/2
  freq/1 -> Add/1
  deg2rad/1 -> sin cos/1

== system sm_stewart_platform/Subsystem/Reference Trajectory Generator3/dz sinusoid ==
  t : Inport
  Add : Sum  Inputs=|++
  Add2 : Sum  Inputs=++|
  amp1 : Gain  Gain=A
  amp2 : Gain  Gain=w*A*pi/180
  deg2rad : Gain  Gain=pi/180
  freq : Gain  Gain=w
  offset : Constant  Value=k  VectorParams1D=off
  phase : Constant  Value=p  VectorParams1D=off
  sin cos : Trigonometry  Operator=sincos
  f : Outport  VectorParamsAs1DForOutWhenUnconnected=off
  f' : Outport  Port=2  VectorParamsAs1DForOutWhenUnconnected=off
  wires:
  t/1 -> freq/1
  Add/1 -> deg2rad/1
  phase/1 -> Add/2
  amp2/1 -> f'/1
  Add2/1 -> f/1
  offset/1 -> Add2/1
  sin cos/1 -> amp1/1
  sin cos/2 -> amp2/1
  amp1/1 -> Add2/2
  freq/1 -> Add/1
  deg2rad/1 -> sin cos/1

== system sm_stewart_platform/Subsystem/Reference Trajectory Generator4/Euler XYZ ==
  angles : Inport
  11 : Fcn  Expr=cos(u[2])*cos(u[3])
  12 : Fcn  Expr=-cos(u[2])*sin(u[3])
  13 : Fcn  Expr=sin(u[2])
  21 : Fcn  Expr=cos(u[3])*sin(u[2])*sin(u[1])+cos(u[1])*sin(u[3])
  22 : Fcn  Expr=cos(u[1])*cos(u[3]) - sin(u[1])*sin(u[2])*sin(u[3])
  23 : Fcn  Expr=-sin(u[1])*cos(u[2])
  31 : Fcn  Expr=sin(u[1])*sin(u[3]) - cos(u[1])*cos(u[3])*sin(u[2])
  32 : Fcn  Expr=cos(u[3])*sin(u[1])+cos(u[1])*sin(u[2])*sin(u[3])
  33 : Fcn  Expr=cos(u[1])*cos(u[2])
  Mux2 : Mux  Inputs=9
  Reshape 9x1->3x3 : Reshape  OutputDimensionality=Customize  OutputDimensions=[3,3]
  R : Outport  VectorParamsAs1DForOutWhenUnconnected=off
  wires:
  angles/1 -> 23/1, 33/1, 13/1, 32/1, 22/1, 12/1, 31/1, 21/1, 11/1
  33/1 -> Mux2/9
  23/1 -> Mux2/8
  13/1 -> Mux2/7
  32/1 -> Mux2/6
  22/1 -> Mux2/5
  12/1 -> Mux2/4
  31/1 -> Mux2/3
  21/1 -> Mux2/2
  11/1 -> Mux2/1
  Mux2/1 -> Reshape 9x1->3x3/1
  Reshape 9x1->3x3/1 -> R/1

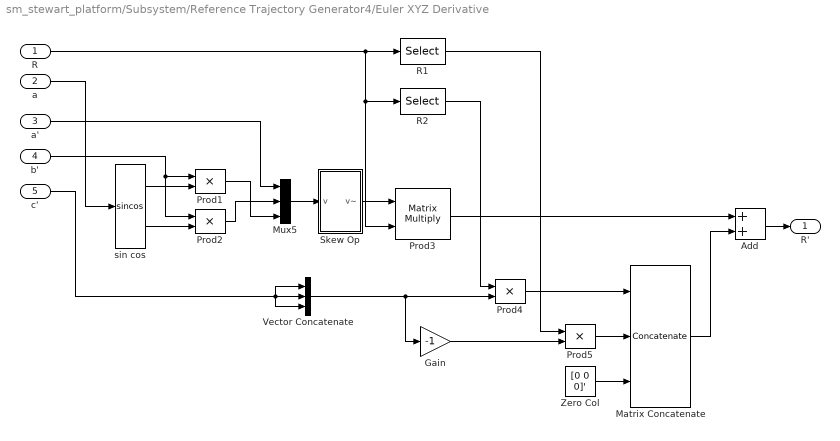
== system sm_stewart_platform/Subsystem/Reference Trajectory Generator4/Euler XYZ Derivative ==
  R : Inport
  a : Inport  Port=2
  a' : Inport  Port=3
  b' : Inport  Port=4
  c' : Inport  Port=5
  Add : Sum
  Gain : Gain  Gain=-1
  Matrix Concatenate : Concatenate  NumInputs=3  Mode=Multidimensional array  ConcatenateDimension=2
  Mux5 : Mux  Inputs=3
  Prod{1..2,4..5} (4 alike) : Product  RndMeth=Zero
  Prod3 : Product  Multiplication=Matrix(*)  RndMeth=Zero
  R1 : Selector  NumberOfDimensions=2  InputPortWidth=3  IndexOptions=Select all,Index vector (dialog)  Indices=[1 3],1  OutputSizes=1,1
  R2 : Selector  NumberOfDimensions=2  InputPortWidth=3  IndexOptions=Select all,Index vector (dialog)  Indices=[1 3],2  OutputSizes=1,1
  Skew Op : Subsystem
  Vector Concatenate : Concatenate  NumInputs=3  Mode=Multidimensional array
  Zero Col : Constant  Value=[0 0 0]'
  sin cos : Trigonometry  Operator=sincos
  R' : Outport  VectorParamsAs1DForOutWhenUnconnected=off
  wires:
  a/1 -> sin cos/1
  sin cos/1 -> Prod1/2
  sin cos/2 -> Prod2/2
  b'/1 -> Prod2/1, Prod1/1
  a'/1 -> Mux5/1
  Prod2/1 -> Mux5/2
  Prod1/1 -> Mux5/3
  Mux5/1 -> Skew Op/1(v)
  Vector Concatenate/1 -> Prod4/2, Gain/1
  R2/1 -> Prod4/1
  Gain/1 -> Prod5/2
  Zero Col/1 -> Matrix Concatenate/3
  Prod5/1 -> Matrix Concatenate/2
  Prod4/1 -> Matrix Concatenate/1
  R1/1 -> Prod5/1
  Prod3/1 -> Add/1
  Matrix Concatenate/1 -> Add/2
  Add/1 -> R'/1
  R/1 -> R1/1, Prod3/2, R2/1
  Skew Op/1(v~) -> Prod3/1
  c'/1 -> Vector Concatenate/2, Vector Concatenate/1, Vector Concatenate/3

== system sm_stewart_platform/Subsystem/Reference Trajectory Generator4/Rx sinusoid ==
  t : Inport
  Add : Sum  Inputs=|++
  Add2 : Sum  Inputs=++|
  amp1 : Gain  Gain=A
  amp2 : Gain  Gain=w*A*pi/180
  deg2rad : Gain  Gain=pi/180
  freq : Gain  Gain=w
  offset : Constant  Value=k  VectorParams1D=off
  phase : Constant  Value=p  VectorParams1D=off
  sin cos : Trigonometry  Operator=sincos
  f : Outport  VectorParamsAs1DForOutWhenUnconnected=off
  f' : Outport  Port=2  VectorParamsAs1DForOutWhenUnconnected=off
  wires:
  t/1 -> freq/1
  Add/1 -> deg2rad/1
  phase/1 -> Add/2
  amp2/1 -> f'/1
  Add2/1 -> f/1
  offset/1 -> Add2/1
  sin cos/1 -> amp1/1
  sin cos/2 -> amp2/1
  amp1/1 -> Add2/2
  freq/1 -> Add/1
  deg2rad/1 -> sin cos/1

== system sm_stewart_platform/Subsystem/Reference Trajectory Generator4/Ry sinusoid ==
  t : Inport
  Add : Sum  Inputs=|++
  Add2 : Sum  Inputs=++|
  amp1 : Gain  Gain=A
  amp2 : Gain  Gain=w*A*pi/180
  deg2rad : Gain  Gain=pi/180
  freq : Gain  Gain=w
  offset : Constant  Value=k  VectorParams1D=off
  phase : Constant  Value=p  VectorParams1D=off
  sin cos : Trigonometry  Operator=sincos
  f : Outport  VectorParamsAs1DForOutWhenUnconnected=off
  f' : Outport  Port=2  VectorParamsAs1DForOutWhenUnconnected=off
  wires:
  t/1 -> freq/1
  Add/1 -> deg2rad/1
  phase/1 -> Add/2
  amp2/1 -> f'/1
  Add2/1 -> f/1
  offset/1 -> Add2/1
  sin cos/1 -> amp1/1
  sin cos/2 -> amp2/1
  amp1/1 -> Add2/2
  freq/1 -> Add/1
  deg2rad/1 -> sin cos/1

== system sm_stewart_platform/Subsystem/Reference Trajectory Generator4/Rz sinusoid ==
  t : Inport
  Add : Sum  Inputs=|++
  Add2 : Sum  Inputs=++|
  amp1 : Gain  Gain=A
  amp2 : Gain  Gain=w*A*pi/180
  deg2rad : Gain  Gain=pi/180
  freq : Gain  Gain=w
  offset : Constant  Value=k  VectorParams1D=off
  phase : Constant  Value=p  VectorParams1D=off
  sin cos : Trigonometry  Operator=sincos
  f : Outport  VectorParamsAs1DForOutWhenUnconnected=off
  f' : Outport  Port=2  VectorParamsAs1DForOutWhenUnconnected=off
  wires:
  t/1 -> freq/1
  Add/1 -> deg2rad/1
  phase/1 -> Add/2
  amp2/1 -> f'/1
  Add2/1 -> f/1
  offset/1 -> Add2/1
  sin cos/1 -> amp1/1
  sin cos/2 -> amp2/1
  amp1/1 -> Add2/2
  freq/1 -> Add/1
  deg2rad/1 -> sin cos/1

== system sm_stewart_platform/Subsystem/Reference Trajectory Generator4/dx sinusoid ==
  t : Inport
  Add : Sum  Inputs=|++
  Add2 : Sum  Inputs=++|
  amp1 : Gain  Gain=A
  amp2 : Gain  Gain=w*A*pi/180
  deg2rad : Gain  Gain=pi/180
  freq : Gain  Gain=w
  offset : Constant  Value=k  VectorParams1D=off
  phase : Constant  Value=p  VectorParams1D=off
  sin cos : Trigonometry  Operator=sincos
  f : Outport  VectorParamsAs1DForOutWhenUnconnected=off
  f' : Outport  Port=2  VectorParamsAs1DForOutWhenUnconnected=off
  wires:
  t/1 -> freq/1
  Add/1 -> deg2rad/1
  phase/1 -> Add/2
  amp2/1 -> f'/1
  Add2/1 -> f/1
  offset/1 -> Add2/1
  sin cos/1 -> amp1/1
  sin cos/2 -> amp2/1
  amp1/1 -> Add2/2
  freq/1 -> Add/1
  deg2rad/1 -> sin cos/1

== system sm_stewart_platform/Subsystem/Reference Trajectory Generator4/dy sinusoid ==
  t : Inport
  Add : Sum  Inputs=|++
  Add2 : Sum  Inputs=++|
  amp1 : Gain  Gain=A
  amp2 : Gain  Gain=w*A*pi/180
  deg2rad : Gain  Gain=pi/180
  freq : Gain  Gain=w
  offset : Constant  Value=k  VectorParams1D=off
  phase : Constant  Value=p  VectorParams1D=off
  sin cos : Trigonometry  Operator=sincos
  f : Outport  VectorParamsAs1DForOutWhenUnconnected=off
  f' : Outport  Port=2  VectorParamsAs1DForOutWhenUnconnected=off
  wires:
  t/1 -> freq/1
  Add/1 -> deg2rad/1
  phase/1 -> Add/2
  amp2/1 -> f'/1
  Add2/1 -> f/1
  offset/1 -> Add2/1
  sin cos/1 -> amp1/1
  sin cos/2 -> amp2/1
  amp1/1 -> Add2/2
  freq/1 -> Add/1
  deg2rad/1 -> sin cos/1

== system sm_stewart_platform/Subsystem/Reference Trajectory Generator4/dz sinusoid ==
  t : Inport
  Add : Sum  Inputs=|++
  Add2 : Sum  Inputs=++|
  amp1 : Gain  Gain=A
  amp2 : Gain  Gain=w*A*pi/180
  deg2rad : Gain  Gain=pi/180
  freq : Gain  Gain=w
  offset : Constant  Value=k  VectorParams1D=off
  phase : Constant  Value=p  VectorParams1D=off
  sin cos : Trigonometry  Operator=sincos
  f : Outport  VectorParamsAs1DForOutWhenUnconnected=off
  f' : Outport  Port=2  VectorParamsAs1DForOutWhenUnconnected=off
  wires:
  t/1 -> freq/1
  Add/1 -> deg2rad/1
  phase/1 -> Add/2
  amp2/1 -> f'/1
  Add2/1 -> f/1
  offset/1 -> Add2/1
  sin cos/1 -> amp1/1
  sin cos/2 -> amp2/1
  amp1/1 -> Add2/2
  freq/1 -> Add/1
  deg2rad/1 -> sin cos/1

== system sm_stewart_platform/Subsystem/Reference Trajectory Generator5/Euler XYZ ==
  angles : Inport
  11 : Fcn  Expr=cos(u[2])*cos(u[3])
  12 : Fcn  Expr=-cos(u[2])*sin(u[3])
  13 : Fcn  Expr=sin(u[2])
  21 : Fcn  Expr=cos(u[3])*sin(u[2])*sin(u[1])+cos(u[1])*sin(u[3])
  22 : Fcn  Expr=cos(u[1])*cos(u[3]) - sin(u[1])*sin(u[2])*sin(u[3])
  23 : Fcn  Expr=-sin(u[1])*cos(u[2])
  31 : Fcn  Expr=sin(u[1])*sin(u[3]) - cos(u[1])*cos(u[3])*sin(u[2])
  32 : Fcn  Expr=cos(u[3])*sin(u[1])+cos(u[1])*sin(u[2])*sin(u[3])
  33 : Fcn  Expr=cos(u[1])*cos(u[2])
  Mux2 : Mux  Inputs=9
  Reshape 9x1->3x3 : Reshape  OutputDimensionality=Customize  OutputDimensions=[3,3]
  R : Outport  VectorParamsAs1DForOutWhenUnconnected=off
  wires:
  angles/1 -> 23/1, 33/1, 13/1, 32/1, 22/1, 12/1, 31/1, 21/1, 11/1
  33/1 -> Mux2/9
  23/1 -> Mux2/8
  13/1 -> Mux2/7
  32/1 -> Mux2/6
  22/1 -> Mux2/5
  12/1 -> Mux2/4
  31/1 -> Mux2/3
  21/1 -> Mux2/2
  11/1 -> Mux2/1
  Mux2/1 -> Reshape 9x1->3x3/1
  Reshape 9x1->3x3/1 -> R/1

== system sm_stewart_platform/Subsystem/Reference Trajectory Generator5/Euler XYZ Derivative ==
  R : Inport
  a : Inport  Port=2
  a' : Inport  Port=3
  b' : Inport  Port=4
  c' : Inport  Port=5
  Add : Sum
  Gain : Gain  Gain=-1
  Matrix Concatenate : Concatenate  NumInputs=3  Mode=Multidimensional array  ConcatenateDimension=2
  Mux5 : Mux  Inputs=3
  Prod{1..2,4..5} (4 alike) : Product  RndMeth=Zero
  Prod3 : Product  Multiplication=Matrix(*)  RndMeth=Zero
  R1 : Selector  NumberOfDimensions=2  InputPortWidth=3  IndexOptions=Select all,Index vector (dialog)  Indices=[1 3],1  OutputSizes=1,1
  R2 : Selector  NumberOfDimensions=2  InputPortWidth=3  IndexOptions=Select all,Index vector (dialog)  Indices=[1 3],2  OutputSizes=1,1
  Skew Op : Subsystem
  Vector Concatenate : Concatenate  NumInputs=3  Mode=Multidimensional array
  Zero Col : Constant  Value=[0 0 0]'
  sin cos : Trigonometry  Operator=sincos
  R' : Outport  VectorParamsAs1DForOutWhenUnconnected=off
  wires:
  a/1 -> sin cos/1
  sin cos/1 -> Prod1/2
  sin cos/2 -> Prod2/2
  b'/1 -> Prod2/1, Prod1/1
  a'/1 -> Mux5/1
  Prod2/1 -> Mux5/2
  Prod1/1 -> Mux5/3
  Mux5/1 -> Skew Op/1(v)
  Vector Concatenate/1 -> Prod4/2, Gain/1
  R2/1 -> Prod4/1
  Gain/1 -> Prod5/2
  Zero Col/1 -> Matrix Concatenate/3
  Prod5/1 -> Matrix Concatenate/2
  Prod4/1 -> Matrix Concatenate/1
  R1/1 -> Prod5/1
  Prod3/1 -> Add/1
  Matrix Concatenate/1 -> Add/2
  Add/1 -> R'/1
  R/1 -> R1/1, Prod3/2, R2/1
  Skew Op/1(v~) -> Prod3/1
  c'/1 -> Vector Concatenate/2, Vector Concatenate/1, Vector Concatenate/3

== system sm_stewart_platform/Subsystem/Reference Trajectory Generator5/Rx sinusoid ==
  t : Inport
  Add : Sum  Inputs=|++
  Add2 : Sum  Inputs=++|
  amp1 : Gain  Gain=A
  amp2 : Gain  Gain=w*A*pi/180
  deg2rad : Gain  Gain=pi/180
  freq : Gain  Gain=w
  offset : Constant  Value=k  VectorParams1D=off
  phase : Constant  Value=p  VectorParams1D=off
  sin cos : Trigonometry  Operator=sincos
  f : Outport  VectorParamsAs1DForOutWhenUnconnected=off
  f' : Outport  Port=2  VectorParamsAs1DForOutWhenUnconnected=off
  wires:
  t/1 -> freq/1
  Add/1 -> deg2rad/1
  phase/1 -> Add/2
  amp2/1 -> f'/1
  Add2/1 -> f/1
  offset/1 -> Add2/1
  sin cos/1 -> amp1/1
  sin cos/2 -> amp2/1
  amp1/1 -> Add2/2
  freq/1 -> Add/1
  deg2rad/1 -> sin cos/1

== system sm_stewart_platform/Subsystem/Reference Trajectory Generator5/Ry sinusoid ==
  t : Inport
  Add : Sum  Inputs=|++
  Add2 : Sum  Inputs=++|
  amp1 : Gain  Gain=A
  amp2 : Gain  Gain=w*A*pi/180
  deg2rad : Gain  Gain=pi/180
  freq : Gain  Gain=w
  offset : Constant  Value=k  VectorParams1D=off
  phase : Constant  Value=p  VectorParams1D=off
  sin cos : Trigonometry  Operator=sincos
  f : Outport  VectorParamsAs1DForOutWhenUnconnected=off
  f' : Outport  Port=2  VectorParamsAs1DForOutWhenUnconnected=off
  wires:
  t/1 -> freq/1
  Add/1 -> deg2rad/1
  phase/1 -> Add/2
  amp2/1 -> f'/1
  Add2/1 -> f/1
  offset/1 -> Add2/1
  sin cos/1 -> amp1/1
  sin cos/2 -> amp2/1
  amp1/1 -> Add2/2
  freq/1 -> Add/1
  deg2rad/1 -> sin cos/1

== system sm_stewart_platform/Subsystem/Reference Trajectory Generator5/Rz sinusoid ==
  t : Inport
  Add : Sum  Inputs=|++
  Add2 : Sum  Inputs=++|
  amp1 : Gain  Gain=A
  amp2 : Gain  Gain=w*A*pi/180
  deg2rad : Gain  Gain=pi/180
  freq : Gain  Gain=w
  offset : Constant  Value=k  VectorParams1D=off
  phase : Constant  Value=p  VectorParams1D=off
  sin cos : Trigonometry  Operator=sincos
  f : Outport  VectorParamsAs1DForOutWhenUnconnected=off
  f' : Outport  Port=2  VectorParamsAs1DForOutWhenUnconnected=off
  wires:
  t/1 -> freq/1
  Add/1 -> deg2rad/1
  phase/1 -> Add/2
  amp2/1 -> f'/1
  Add2/1 -> f/1
  offset/1 -> Add2/1
  sin cos/1 -> amp1/1
  sin cos/2 -> amp2/1
  amp1/1 -> Add2/2
  freq/1 -> Add/1
  deg2rad/1 -> sin cos/1

== system sm_stewart_platform/Subsystem/Reference Trajectory Generator5/dx sinusoid ==
  t : Inport
  Add : Sum  Inputs=|++
  Add2 : Sum  Inputs=++|
  amp1 : Gain  Gain=A
  amp2 : Gain  Gain=w*A*pi/180
  deg2rad : Gain  Gain=pi/180
  freq : Gain  Gain=w
  offset : Constant  Value=k  VectorParams1D=off
  phase : Constant  Value=p  VectorParams1D=off
  sin cos : Trigonometry  Operator=sincos
  f : Outport  VectorParamsAs1DForOutWhenUnconnected=off
  f' : Outport  Port=2  VectorParamsAs1DForOutWhenUnconnected=off
  wires:
  t/1 -> freq/1
  Add/1 -> deg2rad/1
  phase/1 -> Add/2
  amp2/1 -> f'/1
  Add2/1 -> f/1
  offset/1 -> Add2/1
  sin cos/1 -> amp1/1
  sin cos/2 -> amp2/1
  amp1/1 -> Add2/2
  freq/1 -> Add/1
  deg2rad/1 -> sin cos/1

== system sm_stewart_platform/Subsystem/Reference Trajectory Generator5/dy sinusoid ==
  t : Inport
  Add : Sum  Inputs=|++
  Add2 : Sum  Inputs=++|
  amp1 : Gain  Gain=A
  amp2 : Gain  Gain=w*A*pi/180
  deg2rad : Gain  Gain=pi/180
  freq : Gain  Gain=w
  offset : Constant  Value=k  VectorParams1D=off
  phase : Constant  Value=p  VectorParams1D=off
  sin cos : Trigonometry  Operator=sincos
  f : Outport  VectorParamsAs1DForOutWhenUnconnected=off
  f' : Outport  Port=2  VectorParamsAs1DForOutWhenUnconnected=off
  wires:
  t/1 -> freq/1
  Add/1 -> deg2rad/1
  phase/1 -> Add/2
  amp2/1 -> f'/1
  Add2/1 -> f/1
  offset/1 -> Add2/1
  sin cos/1 -> amp1/1
  sin cos/2 -> amp2/1
  amp1/1 -> Add2/2
  freq/1 -> Add/1
  deg2rad/1 -> sin cos/1

== system sm_stewart_platform/Subsystem/Reference Trajectory Generator5/dz sinusoid ==
  t : Inport
  Add : Sum  Inputs=|++
  Add2 : Sum  Inputs=++|
  amp1 : Gain  Gain=A
  amp2 : Gain  Gain=w*A*pi/180
  deg2rad : Gain  Gain=pi/180
  freq : Gain  Gain=w
  offset : Constant  Value=k  VectorParams1D=off
  phase : Constant  Value=p  VectorParams1D=off
  sin cos : Trigonometry  Operator=sincos
  f : Outport  VectorParamsAs1DForOutWhenUnconnected=off
  f' : Outport  Port=2  VectorParamsAs1DForOutWhenUnconnected=off
  wires:
  t/1 -> freq/1
  Add/1 -> deg2rad/1
  phase/1 -> Add/2
  amp2/1 -> f'/1
  Add2/1 -> f/1
  offset/1 -> Add2/1
  sin cos/1 -> amp1/1
  sin cos/2 -> amp2/1
  amp1/1 -> Add2/2
  freq/1 -> Add/1
  deg2rad/1 -> sin cos/1
